simulink model "simulacao_camera"  (R2017a)
settings: Solver=VariableStepAuto  StartTime=0.0  StopTime=10.0  RelTol=1e-3
libraries: simulink x1
settings Model: Creator=dscat  LastModifiedBy=dscat

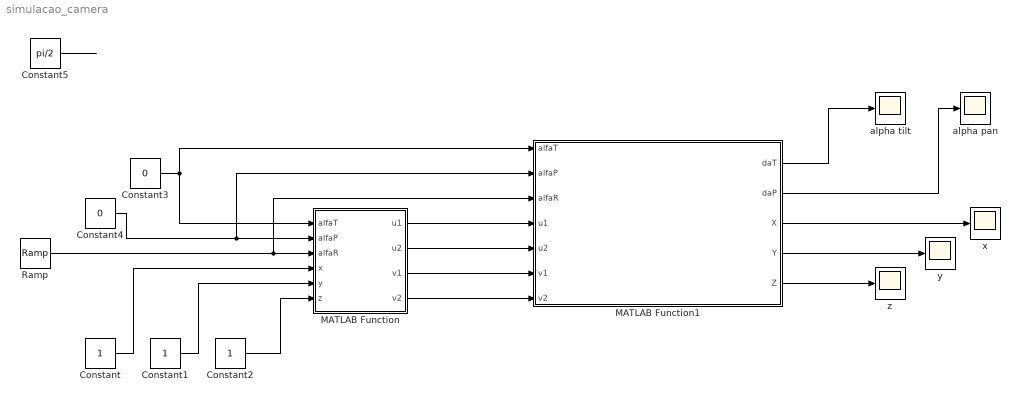
== system simulacao_camera ==
  Constant : Constant
  Constant1 : Constant
  Constant2 : Constant
  Constant3 : Constant  Value=0
  Constant4 : Constant  Value=0
  Constant5 : Constant  Value=pi/2
  MATLAB Function : MATLAB Function  TreatAsAtomicUnit=on
  MATLAB Function1 : MATLAB Function  TreatAsAtomicUnit=on
  Ramp : simulink/Sources/Ramp  slope=pi/12  start=0  X0=0
  alpha pan : Scope
  alpha tilt : Scope
  x : Scope
  y : Scope
  z : Scope
  wires:
  MATLAB Function/4(v2) -> MATLAB Function1/7(v2)
  MATLAB Function/3(v1) -> MATLAB Function1/6(v1)
  MATLAB Function/2(u2) -> MATLAB Function1/5(u2)
  MATLAB Function/1(u1) -> MATLAB Function1/4(u1)
  Constant2/1 -> MATLAB Function/6(z)
  Constant1/1 -> MATLAB Function/5(y)
  Constant/1 -> MATLAB Function/4(x)
  MATLAB Function1/1(daT) -> alpha tilt/1
  MATLAB Function1/2(daP) -> alpha pan/1
  MATLAB Function1/3(X) -> x/1
  MATLAB Function1/4(Y) -> y/1
  MATLAB Function1/5(Z) -> z/1
  Constant5/1 -> ?
  Constant4/1 -> MATLAB Function1/2(alfaP), MATLAB Function/2(alfaP)
  Constant3/1 -> MATLAB Function1/1(alfaT), MATLAB Function/1(alfaT)
  Ramp/1 -> MATLAB Function1/3(alfaR), MATLAB Function/3(alfaR)

== matlab function simulacao_camera/MATLAB Function1 ==
  data: alfaT input; daT output; alfaP input; alfaR input; u1 input; u2 input; v1 input; v2 input; daP output; X output; Y output; Z output
function [daT, daP, X,Y,Z  ] = image2real( alfaT,alfaP,alfaR, u1,u2,v1,v2)
% daT -> Delta Alfa Tilt
% daP -> Delta Alfa Pan
% AlfaR -> Lido dos encoders


l = 0.15; %Tamanho do alvo (m) 
f = 664;

X = (l*(f*cos(alfaP-alfaR) - u2*sin(alfaP-alfaR))*(- cos(alfaP-alfaR)*sin(alfaP-alfaR)*f^2 + (u1 - cos(alfaP-alfaR)^2*(u1 + u2))*f + u1*u2*cos(alfaP-alfaR)*sin(alfaP-alfaR)))/(f*(u2*cos(alfaP-alfaR) + f*sin(alfaP-alfaR))*(u1 - u2));

%  X = (l*(f*cos(alfaT) - v2*sin(alfaT))*(- cos(alfaT)*sin(alfaT)*f^2 + (v1 - cos(alfaT)^2*(v1 + v2))*f + v1*v2*cos(alfaT)*sin(alfaT)))/(f*(f*sin(alfaT) + v2*cos(alfaT))*(v1 - v2));

Y = -(l*(2*cos(alfaP-alfaR)*sin(alfaP-alfaR)*f^2 + (u1 + u2)*(2*cos(alfaP-alfaR)^2 - 1)*f - 2*u1*u2*cos(alfaP-alfaR)*sin(alfaP-alfaR)))/(2*f*(u1 - u2));

Z  = -(l*(2*cos(alfaT)*sin(alfaT)*f^2 + (v1 + v2)*(2*cos(alfaT)^2 - 1)*f - 2*v1*v2*cos(alfaT)*sin(alfaT)))/(2*f*(v1 - v2));
 
daP = double(atan(Y/X)-alfaR);
daT = double(atan(Z/(sqrt((X)^2+(Y)^2))));


end

== matlab function simulacao_camera/MATLAB Function ==
  data: alfaT input; u1 output; alfaP input; alfaR input; x input; y input; z input; u2 output; v1 output; v2 output
function [u1, u2, v1, v2] = real2image(alfaT,alfaP,alfaR,x,y,z)
L = 0.15;
f = 664;
u1 = f*(-sin(alfaP-alfaR)*(-x)+cos(alfaP-alfaR)*((L/2)-y))/((cos(alfaP-alfaR)*(-x)+sin(alfaP-alfaR)*((L/2)-y)));
u2 = f*(-sin(alfaP-alfaR)*(-x)+cos(alfaP-alfaR)*((-L/2)-y))/((cos(alfaP-alfaR)*(-x)+sin(alfaP-alfaR)*((-L/2)-y)));
v1 = f*(-sin(alfaT)*(-x)+cos(alfaT)*((L/2)-z))/((cos(alfaT)*(-x)+sin(alfaT)*((L/2)-z)));
v2 = f*(-sin(alfaT)*(-x)+cos(alfaT)*((-L/2)-z))/((cos(alfaT)*(-x)+sin(alfaT)*((-L/2)-z)));

end
